simulink model "mathModel_v1"  (R2026a)
settings: Solver=VariableStepAuto  StopTime=40
InitFcn:
  | skidpad_init
undefined symbols (not defined in the file): ctrl, ic, skidpad, waypoints
libraries: slpidlib x2, sl_discontinuities x1
settings Model: Creator=lholliday  LastModifiedBy=lholliday

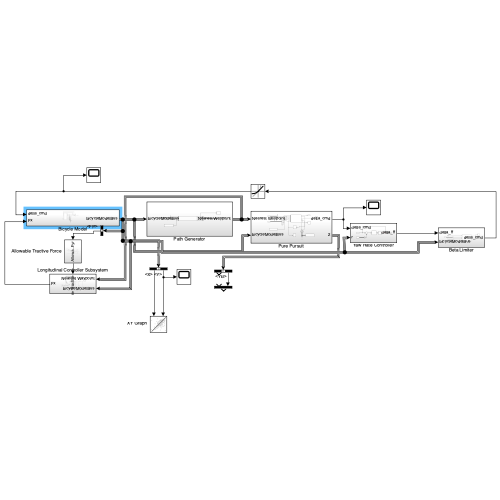
[thumbnail: Simulink's stored preview of the top-level diagram]
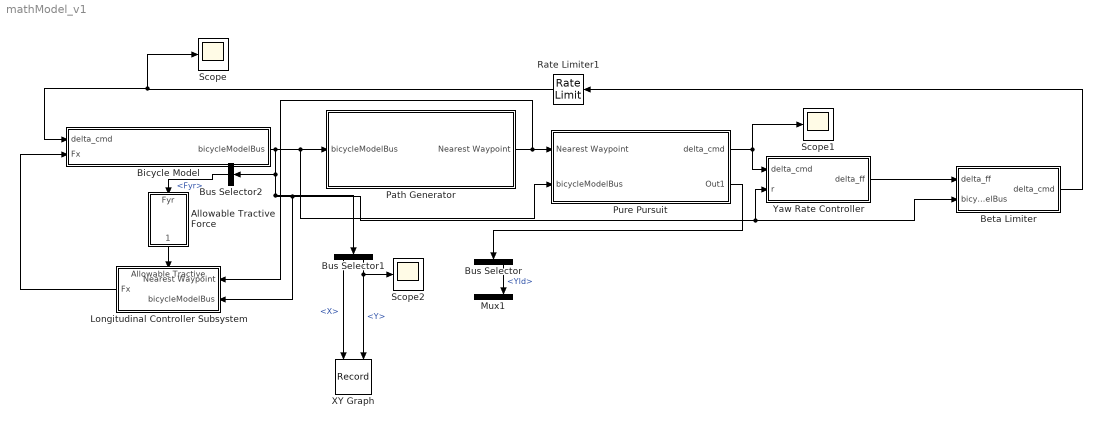
== system mathModel_v1 ==
  Allowable Tractive Force : Subsystem
  Beta Limiter : Subsystem
  Bicycle Model : Subsystem
  Bus Selector : BusSelector  OutputSignals=Xld,Yld
  Bus Selector1 : BusSelector  OutputSignals=X,Y
  Bus Selector2 : BusSelector  OutputSignals=Fyr
  Longitudinal Controller Subsystem : Subsystem
      settings: PortSchema="{\"entries\":[{\"content\":{\"sides\":[{\"content\":{\"connectorIds\":[\"In1\",\"In2\"]},\"type\":\"ConnectorPlacement.EquallySpacedRectSide\",\"uuid\":\"bfc4df2a-5cef-4a02-bb43-7ec6f11f5372\"},{\"content\":{\"connectorIds\":[\"Out1\"],\"side\":\"RIGHT\"},\"type\":\"ConnectorPlacement.EquallySpacedRectSide\",\"uuid\":\"aa21c5e5-626b-425c-a734-c90a404eca5d\"},{\"content\":{\"connectorIds\":[\"In3\"],\"side\":\"TOP\"},\"type\":\"ConnectorPlacement.EquallySpacedRectSide\",\"uuid\":\"e7d9cb0b-dcbc-491d-a1d2-601b886fc6af\"}]},\"type\":\"ConnectorPlacement.EquallySpacedConnector\",\"uuid\":\"7c1271a6-ba3b-4cb7-a1ac-4d930dd7b7e0\"}],\"packageUris\":[\"http://schema.mathworks.com/mf0/Connector/R2020b\"],\"version\":\"1.0\"}"
  Mux1 : Mux  Inputs=2
  Path Generator : Subsystem
  Pure Pursuit : Subsystem
  Rate Limiter1 : RateLimiter  RisingSlewLimit=0.2  FallingSlewLimit=-0.2  SampleTimeMode=inherited
  Scope : Scope
      settings: ActiveDisplayYMinimum=-1  ActiveDisplayYMaximum=1  DataLoggingVariableName=ScopeData8
  Scope1 : Scope
      settings: ActiveDisplayYMinimum=-1.3364775966231448  ActiveDisplayYMaximum=1.4581321408819214  DataLoggingVariableName=ScopeData9
  Scope2 : Scope
      settings: DataLoggingVariableName=ScopeData13
  XY Graph : Record  NumPorts=2.0  FileSettingsInternal="{\"entries\":[{\"content\":{\"excelSettings\":{\"content\":{},\"type\":\"Streamout.ExcelSettings\"},\"parquetSettings\":{\"content\":{},\"type\":\"Streamout.ParquetSettings\"}},\"type\":\"Streamout.FileSettingStorage\",\"uuid\":\"\"}],\"packageUris\":[\"http:\\/\\/schema.mathworks.com\\/mf0\\/streamout_blocks\\/R2020a\"],\"version\":\"1.0\"}"  FrameSettings=[0, 0]  Layout=[1 1]  SignalsInternal="{\"entries\":[{\"content\":{\"signals\":[{\"content\":{\"blockPath\":[],\"dimensions\":[1],\"domain\":\"\",\"lineColor\":\"#a2142f\",\"plots\":[ 1 ],\"port\":1,\"signalID\":1,\"signalName\":\"<X>\"},\"type\":\"RecordBlkView.Signal\",\"uuid\":\"\"},{\"content\":{\"blockPath\":[],\"dimensions\":[1],\"domain\":\"\",\"lineColor\":\"#139fff\",\"plots\":[ 1 ],\"port\":2,\"signalID\":2,\"signalName\":\"<Y>\"},\"type\":\"RecordBlkView.Signal\",\"uuid\":\"\"}]},\"type\":\"RecordBlkView.InputSignals\",\"uuid\":\"\"}],\"packageUris\":[\"http:\\/\\/schema.mathworks.com\\/mf0\\/streamout_blocks\\/R2020a\"],\"version\":\"1.0\"}"  VisualizationBindings="{\"xyplotplugin\":{\"info\":[{\"series\":[{\"bindingParametersList\":[{\"parameter\":\"X-Axis\",\"signalID\":1,\"signalName\":\"<X>\"},{\"parameter\":\"Y-Axis\",\"signalID\":2,\"signalName\":\"<Y>\"}],\"seriesID\":0}],\"subplotID\":1}]}}"  CompatibilityTag=XY
  Yaw Rate Controller : Subsystem
  wires:
  Path Generator/1(Nearest Waypoint) -> Longitudinal Controller Subsystem/1(Nearest Waypoint), Pure Pursuit/1(Nearest Waypoint)
  Bicycle Model/1(bicycleModelBus) -> Path Generator/1(bicycleModelBus), Pure Pursuit/2(bicycleModelBus), Longitudinal Controller Subsystem/2(bicycleModelBus), Beta Limiter/2(bicycleModelBus), Yaw Rate Controller/2(r), Bus Selector1/1, Bus Selector2/1
  Beta Limiter/1(delta_cmd) -> Rate Limiter1/1
  Longitudinal Controller Subsystem/1(Fx) -> Bicycle Model/2(Fx)
  Pure Pursuit/1(delta_cmd) -> Yaw Rate Controller/1(delta_cmd), Scope1/1
  Yaw Rate Controller/1(delta_ff) -> Beta Limiter/1(delta_ff)
  Pure Pursuit/2(Out1) -> Bus Selector/1
  Bus Selector/2 -> Mux1/2  "<Yld>"
  Bus Selector1/1 -> XY Graph/1  "<X>"
  Bus Selector1/2 -> Scope2/1, XY Graph/2  "<Y>"
  Rate Limiter1/1 -> Scope/1, Bicycle Model/1(delta_cmd)
  Allowable Tractive Force/1(Allowable Tractive) -> Longitudinal Controller Subsystem/3(Allowable Tractive)
  Bus Selector2/1 -> Allowable Tractive Force/1(Fyr)  "<Fyr>"

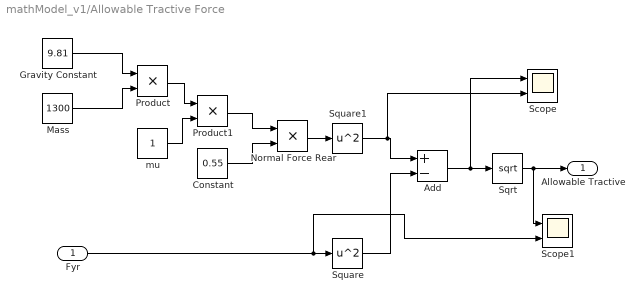
== system mathModel_v1/Allowable Tractive Force ==
  Fyr : Inport
  Add : Sum  Inputs=+-
  Constant : Constant  Value=0.55
  Gravity Constant : Constant  Value=9.81
  Mass : Constant  Value=1300
  Normal Force Rear : Product
  Product : Product
  Product1 : Product
  Scope : Scope  NumInputPorts=2
      settings: ActiveDisplayYMinimum=-2.6445905173405474E+6  ActiveDisplayYMaximum=5.4958621415815629E+7  DataLoggingVariableName=ScopeData17
  Scope1 : Scope  NumInputPorts=2
      settings: ActiveDisplayYMinimum=1109.0174008180957  ActiveDisplayYMaximum=7670.2758443535458  DataLoggingVariableName=ScopeData18
  Sqrt : Sqrt
  Square : Math  Operator=square
  Square1 : Math  Operator=square
  mu : Constant
  Allowable Tractive : Outport
  wires:
  Fyr/1 -> Scope1/2, Square/1
  Mass/1 -> Product/2
  Gravity Constant/1 -> Product/1
  mu/1 -> Product1/2
  Product/1 -> Product1/1
  Constant/1 -> Normal Force Rear/2
  Product1/1 -> Normal Force Rear/1
  Square/1 -> Add/2
  Normal Force Rear/1 -> Square1/1
  Square1/1 -> Scope/2, Add/1
  Add/1 -> Scope/1, Sqrt/1
  Sqrt/1 -> Scope1/1, Allowable Tractive/1

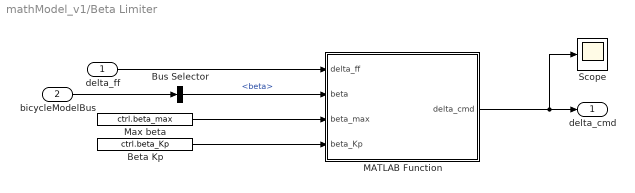
== system mathModel_v1/Beta Limiter ==
  delta_ff : Inport
  bicycleModelBus : Inport  Port=2
  Beta Kp : Constant  Value=ctrl.beta_Kp
  Bus Selector : BusSelector  OutputSignals=beta
  MATLAB Function : MATLAB Function  TreatAsAtomicUnit=on
  Max beta : Constant  Value=ctrl.beta_max
  Scope : Scope
      settings: ActiveDisplayYMinimum=-1.1215665093165463  ActiveDisplayYMaximum=1.1329055665670569  DataLoggingVariableName=ScopeData11
  delta_cmd : Outport
  wires:
  bicycleModelBus/1 -> Bus Selector/1
  delta_ff/1 -> MATLAB Function/1(delta_ff)
  Bus Selector/1 -> MATLAB Function/2(beta)  "<beta>"
  MATLAB Function/1(delta_cmd) -> delta_cmd/1, Scope/1
  Max beta/1 -> MATLAB Function/3(beta_max)
  Beta Kp/1 -> MATLAB Function/4(beta_Kp)

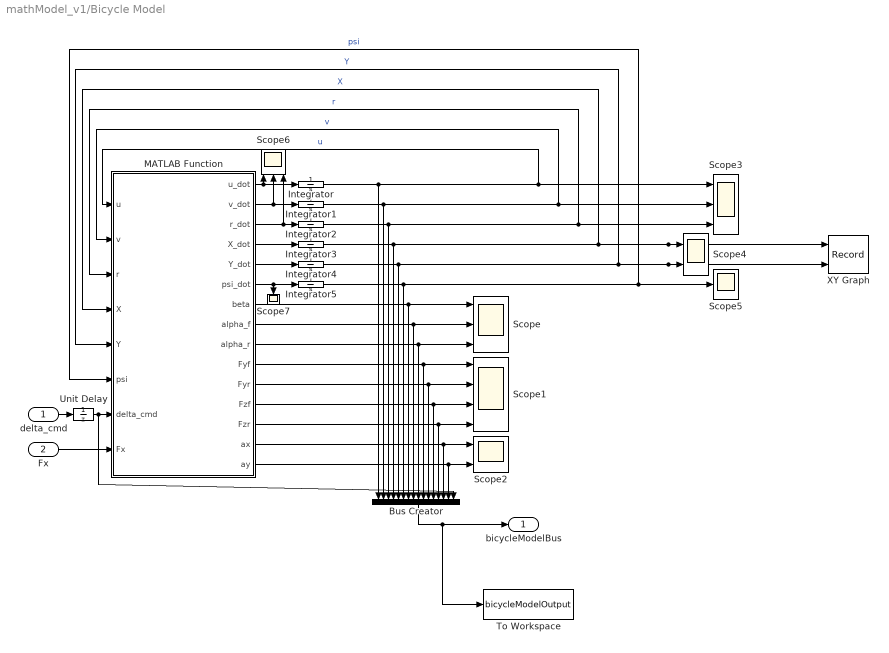
== system mathModel_v1/Bicycle Model ==
  delta_cmd : Inport
  Fx : Inport  Port=2
  Bus Creator : BusCreator  Inputs=16
  Integrator : Integrator  InitialCondition=1
  Integrator1 : Integrator
  Integrator2 : Integrator
  Integrator3 : Integrator  InitialCondition=ic.X
  Integrator4 : Integrator  InitialCondition=ic.Y
  Integrator5 : Integrator
  MATLAB Function : MATLAB Function  TreatAsAtomicUnit=on
  Scope : Scope  NumInputPorts=3
      settings: ActiveDisplayYMinimum=-3.8834487978477066  ActiveDisplayYMaximum=5.2081564111480709
  Scope1 : Scope  NumInputPorts=4
      settings: ActiveDisplayYMinimum=-1  ActiveDisplayYMaximum=1
  Scope2 : Scope  NumInputPorts=2
      settings: ActiveDisplayYMinimum=-1  ActiveDisplayYMaximum=1  DataLoggingVariableName=ScopeData2
  Scope3 : Scope  NumInputPorts=3
      settings: ActiveDisplayYMinimum=-3.5254490278371251  ActiveDisplayYMaximum=31.729041250534134  DataLoggingVariableName=ScopeData3
  Scope4 : Scope  NumInputPorts=2
      settings: ActiveDisplayYMinimum=-1031.663648785918  ActiveDisplayYMaximum=2103.4580897021219  DataLoggingVariableName=ScopeData4
  Scope5 : Scope
      settings: ActiveDisplayYMinimum=-1  ActiveDisplayYMaximum=1  DataLoggingVariableName=ScopeData5
  Scope6 : Scope  NumInputPorts=3
      settings: ActiveDisplayYMinimum=-1.4708935468625282  ActiveDisplayYMaximum=6.1584326163180583  DataLoggingVariableName=ScopeData6
  Scope7 : Scope
      settings: ActiveDisplayYMinimum=-1.109696536806452  ActiveDisplayYMaximum=1.2916224827655673  DataLoggingVariableName=ScopeData10
  To Workspace : ToWorkspace  VariableName=bicycleModelOutput  SaveFormat=Timeseries  SampleTime=-1
  Unit Delay : UnitDelay  SampleTime=-1
  XY Graph : Record  NumPorts=2.0  FileSettingsInternal="{\"entries\":[{\"content\":{\"excelSettings\":{\"content\":{},\"type\":\"Streamout.ExcelSettings\"},\"parquetSettings\":{\"content\":{},\"type\":\"Streamout.ParquetSettings\"}},\"type\":\"Streamout.FileSettingStorage\",\"uuid\":\"\"}],\"packageUris\":[\"http:\\/\\/schema.mathworks.com\\/mf0\\/streamout_blocks\\/R2020a\"],\"version\":\"1.0\"}"  FrameSettings=[0, 0]  Layout=[1 1]  SignalsInternal="{\"entries\":[{\"content\":{\"signals\":[{\"content\":{\"blockPath\":[],\"dimensions\":[1],\"domain\":\"\",\"lineColor\":\"#a2142f\",\"plots\":[ 1 ],\"port\":1,\"signalID\":1,\"signalName\":\"X\"},\"type\":\"RecordBlkView.Signal\",\"uuid\":\"\"},{\"content\":{\"blockPath\":[],\"dimensions\":[1],\"domain\":\"\",\"lineColor\":\"#139fff\",\"plots\":[ 1 ],\"port\":2,\"signalID\":2,\"signalName\":\"Y\"},\"type\":\"RecordBlkView.Signal\",\"uuid\":\"\"}]},\"type\":\"RecordBlkView.InputSignals\",\"uuid\":\"\"}],\"packageUris\":[\"http:\\/\\/schema.mathworks.com\\/mf0\\/streamout_blocks\\/R2020a\"],\"version\":\"1.0\"}"  VisualizationBindings="{\"xyplotplugin\":{\"info\":[{\"series\":[{\"bindingParametersList\":[{\"parameter\":\"X-Axis\",\"signalID\":1,\"signalName\":\"X\"},{\"parameter\":\"Y-Axis\",\"signalID\":2,\"signalName\":\"Y\"}],\"seriesID\":0}],\"subplotID\":1}]}}"  CompatibilityTag=XY
  bicycleModelBus : Outport
  wires:
  ? -> ?
  MATLAB Function/2(v_dot) -> Scope6/2, Integrator1/1
  MATLAB Function/3(r_dot) -> Scope6/3, Integrator2/1
  MATLAB Function/4(X_dot) -> Integrator3/1
  MATLAB Function/5(Y_dot) -> Integrator4/1
  MATLAB Function/6(psi_dot) -> Scope7/1, Integrator5/1
  MATLAB Function/1(u_dot) -> Scope6/1, Integrator/1
  Integrator1/1 -> Scope3/2, MATLAB Function/2(v), Bus Creator/2  "v"
  Integrator2/1 -> Scope3/3, MATLAB Function/3(r), Bus Creator/3  "r"
  Integrator3/1 -> MATLAB Function/4(X), XY Graph/1, Scope4/1, Bus Creator/4  "X"
  Integrator4/1 -> MATLAB Function/5(Y), XY Graph/2, Scope4/2, Bus Creator/5  "Y"
  Integrator5/1 -> MATLAB Function/6(psi), Scope5/1, Bus Creator/6  "psi"
  MATLAB Function/8(alpha_f) -> Scope/2, Bus Creator/8
  MATLAB Function/7(beta) -> Scope/1, Bus Creator/7
  MATLAB Function/9(alpha_r) -> Scope/3, Bus Creator/9
  MATLAB Function/10(Fyf) -> Scope1/1, Bus Creator/10
  MATLAB Function/11(Fyr) -> Scope1/2, Bus Creator/11
  MATLAB Function/12(Fzf) -> Scope1/3, Bus Creator/12
  MATLAB Function/13(Fzr) -> Scope1/4, Bus Creator/13
  MATLAB Function/15(ay) -> Scope2/2, Bus Creator/15
  MATLAB Function/14(ax) -> Scope2/1, Bus Creator/14
  Fx/1 -> MATLAB Function/8(Fx)
  Bus Creator/1 -> To Workspace/1, bicycleModelBus/1
  Integrator/1 -> Scope3/1, MATLAB Function/1(u), Bus Creator/1  "u"
  delta_cmd/1 -> Unit Delay/1
  Unit Delay/1 -> Bus Creator/16, MATLAB Function/7(delta_cmd)

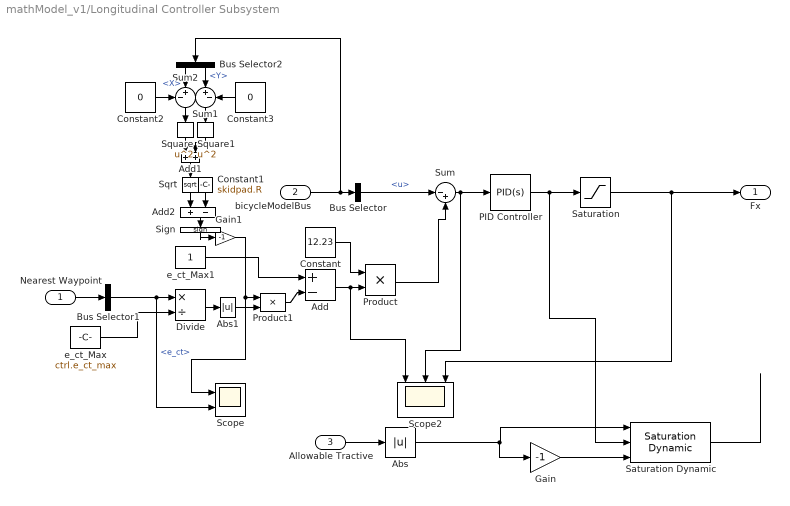
== system mathModel_v1/Longitudinal Controller Subsystem ==
  Nearest Waypoint : Inport
  bicycleModelBus : Inport  Port=2
  Allowable Tractive : Inport  Port=3
  Abs : Abs  SaturateOnIntegerOverflow=off
  Abs1 : Abs  SaturateOnIntegerOverflow=off
  Add : Sum  Inputs=+-
  Add1 : Sum
  Add2 : Sum  Inputs=+-
  Bus Selector : BusSelector  OutputSignals=u
  Bus Selector1 : BusSelector  OutputSignals=e_ct
  Bus Selector2 : BusSelector  OutputSignals=X,Y
  Constant : Constant  Value=12.23
  Constant1 : Constant  Value=skidpad.R
  Constant2 : Constant  Value=0
  Constant3 : Constant  Value=0
  Divide : Product  Inputs=*/
  Gain : Gain  Gain=-1
  Gain1 : Gain  Gain=-1
  PID Controller : slpidlib/PID Controller  Controller=PID  Form=Parallel  TimeDomain=Continuous-time  UseExternalTs=off  SampleTime=-1  IntegratorMethod=Forward Euler  FilterMethod=Forward Euler  ControllerParametersSource=internal  P=ctrl.spd_Kp  I=ctrl.spd_Ki  UseKiTs=off  D=ctrl.spd_Kd  UseExternalDerivativeSource=off  N=100  UseFilter=on  TunerSelectOption=Transfer Function Based (PID Tuner App)  InitialConditionSource=internal  InitialConditionForIntegrator=0  InitialConditionForFilter=0  DifferentiatorICPrevScaledInput=0  ExternalReset=none  TrackingMode=off  Kt=1  LimitOutput=off  SatLimitsSource=internal  UpperSaturationLimit=inf  LowerSaturationLimit=-inf  LinearizeAsGain=on  AntiWindupMode=none  Kb=1  LimitIntegrator=off  UpperIntegratorSaturationLimit=inf  LowerIntegratorSaturationLimit=-inf  POutMin=[]  POutMax=[]  IOutMin=[]  IOutMax=[]  DOutMin=[]  DOutMax=[]  NOutMin=[]  NOutMax=[]  SumOutMin=[]  SumOutMax=[]  SaturationOutMin=[]  SaturationOutMax=[]  PParamMin=[]  PParamMax=[]  IParamMin=[]  IParamMax=[]  DParamMin=[]  DParamMax=[]  NParamMin=[]  NParamMax=[]  KbParamMin=[]  KbParamMax=[]  KtParamMin=[]  KtParamMax=[]  KbOutMin=[]  KbOutMax=[]  KtOutMin=[]  KtOutMax=[]  IntegratorOutMin=[]  IntegratorOutMax=[]  FilterOutMin=[]  FilterOutMax=[]  SumI1OutMin=[]  SumI1OutMax=[]  SumI2OutMin=[]  SumI2OutMax=[]  SumI3OutMin=[]  SumI3OutMax=[]  SumI4OutMin=[]  SumI4OutMax=[]  SumDOutMin=[]  SumDOutMax=[]  DifferentiatorOutMin=[]  DifferentiatorOutMax=[]  FilterDiffOutCoefMin=[]  FilterDiffOutCoefMax=[]  ReciprocalOutMin=[]  ReciprocalOutMax=[]  SumDenOutMin=[]  SumDenOutMax=[]  SumNumOutMin=[]  SumNumOutMax=[]  DivideOutMin=[]  DivideOutMax=[]  UdiffTsProdOutMin=[]  UdiffTsProdOutMax=[]  NTsProdOutMin=[]  NTsProdOutMax=[]  UintegralTsProdOutMin=[]  UintegralTsProdOutMax=[]  UngainTsProdOutMin=[]  UngainTsProdOutMax=[]  ClampingZeroOutDataTypeStr=Inherit: Inherit via back propagation  ClampingZeroOutMin=[]  ClampingZeroOutMax=[]  FilterDenConstantOutDataTypeStr=Inherit: Inherit via back propagation  FilterDenConstantOutMin=[]  FilterDenConstantOutMax=[]  PCopyOutDataTypeStr=Inherit: Inherit via back propagation  PCopyOutMin=[]  PCopyOutMax=[]  NCopyOutDataTypeStr=Inherit: Inherit via back propagation  NCopyOutMin=[]  NCopyOutMax=[]  IntegratorContinuousStateAttributes=''  IntegratorStateMustResolveToSignalObject=off  IntegratorRTWStateStorageClass=Auto  FilterContinuousStateAttributes=''  FilterStateMustResolveToSignalObject=off  FilterRTWStateStorageClass=Auto  ParallelPVariant=InternalParameters  IdealPVariant=Disabled  IVariant=InternalParameters  DVariant=InternalParameters  IntegratorVariant=Continuous  SatVariant=Disabled  AWVariant=Passthrough  PCopyVariant=Disabled  TRVariant=Disabled  FdbkBlocksVariant=Forward  IdealPFdbkVariant=Disabled  SatFdbkVariant=Disabled  DerivativeFilterVariant=ContFilter  NVariant=InternalParameters  NCopyVariant=Disabled  FilterICVariant=InternalICsFilter  IntegratorICVariant=InternalICs  ExternalResetVariant=Disabled  TRSumVariant=Passthrough  SumFdbkVariant=Disabled  SumVariant=Sum_PID  TsampFilterVariant=InternalTs  TsampNgainVariant=Passthrough  TsampIntegralVariant=Disabled_SignalSpec  ExternalSaturationOutDataTypeStr=Inherit: Same as second input  DerivativeSourceVariant=ErrorSignal  PreIntVariant=InternalPreInt
  Product : Product
  Product1 : Product
  Saturation : Saturate  UpperLimit=ctrl.Fx_max  LowerLimit=ctrl.Fx_min
  Saturation Dynamic : sl_discontinuities/Saturation Dynamic  OutMin=[]  OutMax=[]  OutDataTypeStr=Inherit: Same as second input  OutDataType=fixdt(1, 16)  OutScaling=2^-10  DoSatur=off
      settings: LibrarySourceBlock=|
      | simulink/Discontinuities/Saturation
      | Dynamic
  Scope : Scope  NumInputPorts=2
      settings: ActiveDisplayYMinimum=-48.92468742696137  ActiveDisplayYMaximum=48.607667503868036  DataLoggingVariableName=ScopeData16
  Scope2 : Scope  NumInputPorts=3
      settings: ActiveDisplayYMinimum=-0.082162988080077839  ActiveDisplayYMaximum=1.1202403320088976  DataLoggingVariableName=ScopeData19
  Sign : Signum
  Sqrt : Sqrt
  Square : Math  Operator=square
  Square1 : Math  Operator=square
  Sum : Sum  Inputs=|-+
  Sum1 : Sum  Inputs=|+-
  Sum2 : Sum  Inputs=-+|
  e_ct_Max : Constant  Value=ctrl.e_ct_max
  e_ct_Max1 : Constant
  Fx : Outport
  wires:
  bicycleModelBus/1 -> Bus Selector/1, Bus Selector2/1
  Sum/1 -> PID Controller/1, Scope2/2
  PID Controller/1 -> Saturation/1, Saturation Dynamic/2
  Saturation/1 -> Scope2/3, Fx/1
  Allowable Tractive/1 -> Abs/1
  Abs/1 -> Gain/1, Saturation Dynamic/1
  Gain/1 -> Saturation Dynamic/3
  Saturation Dynamic/1 -> ?
  Nearest Waypoint/1 -> Bus Selector1/1
  Bus Selector1/1 -> Scope/2, Divide/1  "<e_ct>"
  e_ct_Max/1 -> Divide/2
  Divide/1 -> Abs1/1
  Product/1 -> Sum/2
  e_ct_Max1/1 -> Add/1
  Add/1 -> Scope2/1, Product/2
  Bus Selector/1 -> Sum/1  "<u>"
  Constant/1 -> Product/1
  Square/1 -> Add1/1
  Square1/1 -> Add1/2
  Add1/1 -> Sqrt/1
  Sqrt/1 -> Add2/1
  Constant1/1 -> Add2/2
  Add2/1 -> Sign/1
  Abs1/1 -> Product1/2
  Sign/1 -> Gain1/1
  Product1/1 -> Add/2
  Constant3/1 -> Sum1/2
  Bus Selector2/2 -> Sum1/1  "<Y>"
  Sum1/1 -> Square1/1
  Sum2/1 -> Square/1
  Bus Selector2/1 -> Sum2/2  "<X>"
  Constant2/1 -> Sum2/1
  Gain1/1 -> Scope/1, Product1/1

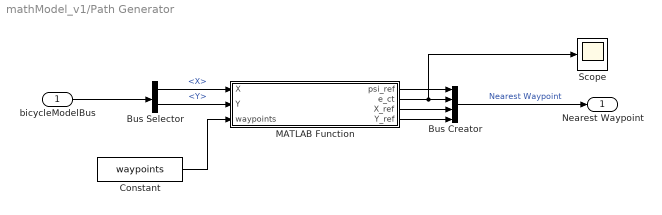
== system mathModel_v1/Path Generator ==
  bicycleModelBus : Inport
  Bus Creator : BusCreator  Inputs=4
  Bus Selector : BusSelector  OutputSignals=X,Y
  Constant : Constant  Value=waypoints
  MATLAB Function : MATLAB Function  TreatAsAtomicUnit=on
  Scope : Scope
      settings: ActiveDisplayYMinimum=-362.12936641992621  ActiveDisplayYMaximum=253.81612411681579  DataLoggingVariableName=ScopeData7
  Nearest Waypoint : Outport
  wires:
  bicycleModelBus/1 -> Bus Selector/1
  Bus Selector/1 -> MATLAB Function/1(X)  "<X>"
  Bus Selector/2 -> MATLAB Function/2(Y)  "<Y>"
  MATLAB Function/1(psi_ref) -> Bus Creator/1
  MATLAB Function/2(e_ct) -> Scope/1, Bus Creator/2
  MATLAB Function/3(X_ref) -> Bus Creator/3
  MATLAB Function/4(Y_ref) -> Bus Creator/4
  Bus Creator/1 -> Nearest Waypoint/1  "Nearest Waypoint"
  Constant/1 -> MATLAB Function/3(waypoints)

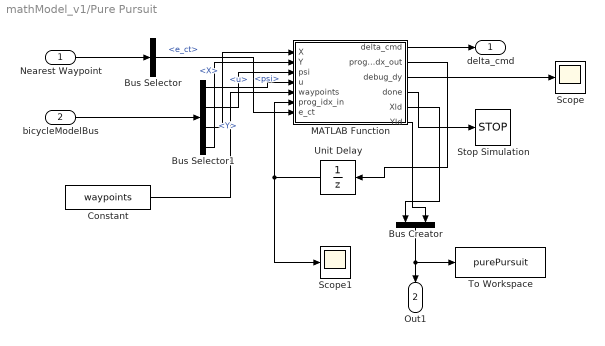
== system mathModel_v1/Pure Pursuit ==
  Nearest Waypoint : Inport
  bicycleModelBus : Inport  Port=2
  Bus Creator : BusCreator  Inputs=2
  Bus Selector : BusSelector  OutputSignals=e_ct
  Bus Selector1 : BusSelector  OutputSignals=u,psi,X,Y
  Constant : Constant  Value=waypoints
  MATLAB Function : MATLAB Function  TreatAsAtomicUnit=on
  Scope : Scope
      settings: ActiveDisplayYMinimum=-282.00787938495415  ActiveDisplayYMaximum=340.50274168342952  DataLoggingVariableName=ScopeData12
  Scope1 : Scope
      settings: ActiveDisplayYMinimum=-19.874999999999996  ActiveDisplayYMaximum=188.875  DataLoggingVariableName=ScopeData14
  Stop Simulation : Stop
  To Workspace : ToWorkspace  VariableName=purePursuit  SaveFormat=Timeseries  SampleTime=-1
  Unit Delay : UnitDelay  InitialCondition=1  SampleTime=0.01
  delta_cmd : Outport
  Out1 : Outport  Port=2
  wires:
  bicycleModelBus/1 -> Bus Selector1/1
  Nearest Waypoint/1 -> Bus Selector/1
  Bus Selector1/1 -> MATLAB Function/4(u)  "<u>"
  Bus Selector1/2 -> MATLAB Function/3(psi)  "<psi>"
  MATLAB Function/1(delta_cmd) -> delta_cmd/1
  Bus Selector1/3 -> MATLAB Function/1(X)  "<X>"
  Bus Selector1/4 -> MATLAB Function/2(Y)  "<Y>"
  Constant/1 -> MATLAB Function/5(waypoints)
  MATLAB Function/3(debug_dy) -> Scope/1
  MATLAB Function/2(prog_idx_out) -> Unit Delay/1
  Unit Delay/1 -> MATLAB Function/6(prog_idx_in), Scope1/1
  MATLAB Function/4(done) -> Stop Simulation/1
  Bus Creator/1 -> To Workspace/1, Out1/1
  MATLAB Function/5(Xld) -> Bus Creator/1
  MATLAB Function/6(Yld) -> Bus Creator/2
  Bus Selector/1 -> MATLAB Function/7(e_ct)  "<e_ct>"

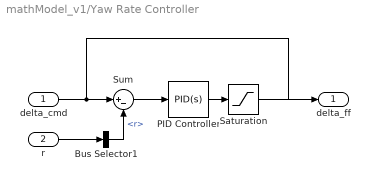
== system mathModel_v1/Yaw Rate Controller ==
  delta_cmd : Inport
  r : Inport  Port=2
  Bus Selector1 : BusSelector  OutputSignals=r
  PID Controller : slpidlib/PID Controller  Controller=PID  Form=Parallel  TimeDomain=Continuous-time  UseExternalTs=off  SampleTime=-1  IntegratorMethod=Forward Euler  FilterMethod=Forward Euler  ControllerParametersSource=internal  P=0.3  I=0.05  UseKiTs=off  D=0  UseExternalDerivativeSource=off  N=100  UseFilter=on  TunerSelectOption=Transfer Function Based (PID Tuner App)  InitialConditionSource=internal  InitialConditionForIntegrator=0  InitialConditionForFilter=0  DifferentiatorICPrevScaledInput=0  ExternalReset=none  TrackingMode=off  Kt=1  LimitOutput=off  SatLimitsSource=internal  UpperSaturationLimit=inf  LowerSaturationLimit=-inf  LinearizeAsGain=on  AntiWindupMode=none  Kb=1  LimitIntegrator=off  UpperIntegratorSaturationLimit=inf  LowerIntegratorSaturationLimit=-inf  POutMin=[]  POutMax=[]  IOutMin=[]  IOutMax=[]  DOutMin=[]  DOutMax=[]  NOutMin=[]  NOutMax=[]  SumOutMin=[]  SumOutMax=[]  SaturationOutMin=[]  SaturationOutMax=[]  PParamMin=[]  PParamMax=[]  IParamMin=[]  IParamMax=[]  DParamMin=[]  DParamMax=[]  NParamMin=[]  NParamMax=[]  KbParamMin=[]  KbParamMax=[]  KtParamMin=[]  KtParamMax=[]  KbOutMin=[]  KbOutMax=[]  KtOutMin=[]  KtOutMax=[]  IntegratorOutMin=[]  IntegratorOutMax=[]  FilterOutMin=[]  FilterOutMax=[]  SumI1OutMin=[]  SumI1OutMax=[]  SumI2OutMin=[]  SumI2OutMax=[]  SumI3OutMin=[]  SumI3OutMax=[]  SumI4OutMin=[]  SumI4OutMax=[]  SumDOutMin=[]  SumDOutMax=[]  DifferentiatorOutMin=[]  DifferentiatorOutMax=[]  FilterDiffOutCoefMin=[]  FilterDiffOutCoefMax=[]  ReciprocalOutMin=[]  ReciprocalOutMax=[]  SumDenOutMin=[]  SumDenOutMax=[]  SumNumOutMin=[]  SumNumOutMax=[]  DivideOutMin=[]  DivideOutMax=[]  UdiffTsProdOutMin=[]  UdiffTsProdOutMax=[]  NTsProdOutMin=[]  NTsProdOutMax=[]  UintegralTsProdOutMin=[]  UintegralTsProdOutMax=[]  UngainTsProdOutMin=[]  UngainTsProdOutMax=[]  ClampingZeroOutDataTypeStr=Inherit: Inherit via back propagation  ClampingZeroOutMin=[]  ClampingZeroOutMax=[]  FilterDenConstantOutDataTypeStr=Inherit: Inherit via back propagation  FilterDenConstantOutMin=[]  FilterDenConstantOutMax=[]  PCopyOutDataTypeStr=Inherit: Inherit via back propagation  PCopyOutMin=[]  PCopyOutMax=[]  NCopyOutDataTypeStr=Inherit: Inherit via back propagation  NCopyOutMin=[]  NCopyOutMax=[]  IntegratorContinuousStateAttributes=''  IntegratorStateMustResolveToSignalObject=off  IntegratorRTWStateStorageClass=Auto  FilterContinuousStateAttributes=''  FilterStateMustResolveToSignalObject=off  FilterRTWStateStorageClass=Auto  ParallelPVariant=InternalParameters  IdealPVariant=Disabled  IVariant=InternalParameters  DVariant=InternalParameters  IntegratorVariant=Continuous  SatVariant=Disabled  AWVariant=Passthrough  PCopyVariant=Disabled  TRVariant=Disabled  FdbkBlocksVariant=Forward  IdealPFdbkVariant=Disabled  SatFdbkVariant=Disabled  DerivativeFilterVariant=ContFilter  NVariant=InternalParameters  NCopyVariant=Disabled  FilterICVariant=InternalICsFilter  IntegratorICVariant=InternalICs  ExternalResetVariant=Disabled  TRSumVariant=Passthrough  SumFdbkVariant=Disabled  SumVariant=Sum_PID  TsampFilterVariant=InternalTs  TsampNgainVariant=Passthrough  TsampIntegralVariant=Disabled_SignalSpec  ExternalSaturationOutDataTypeStr=Inherit: Same as second input  DerivativeSourceVariant=ErrorSignal  PreIntVariant=InternalPreInt
  Saturation : Saturate  UpperLimit=30*pi()/180  LowerLimit=- 30*pi()/180
  Sum : Sum  Inputs=|+-
  delta_ff : Outport
  wires:
  r/1 -> Bus Selector1/1
  Sum/1 -> PID Controller/1
  Bus Selector1/1 -> Sum/2  "<r>"
  PID Controller/1 -> Saturation/1
  Saturation/1 -> ?
  delta_cmd/1 -> delta_ff/1, Sum/1

== matlab function mathModel_v1/Path Generator/MATLAB Function ==
  data: X input; psi_ref output; Y input; e_ct output; X_ref output; Y_ref output; waypoints input
function [psi_ref, e_ct, X_ref, Y_ref] = nearest_waypoint(X, Y, waypoints)

% Find nearest waypoint
dx   = waypoints(:,1) - X;
dy   = waypoints(:,2) - Y;
dist = sqrt(dx.^2 + dy.^2);
[~, idx] = min(dist);

psi_ref = waypoints(idx, 3);
X_ref   = waypoints(idx, 1);
Y_ref   = waypoints(idx, 2);

dx_ref = X - X_ref;
dy_ref = Y - Y_ref;
e_ct   = -sin(psi_ref)*dx_ref + cos(psi_ref)*dy_ref;

== matlab function mathModel_v1/Bicycle Model/MATLAB Function ==
  data: u_dot output; v_dot output; u input; v input; r_dot output; X_dot output; r input; X input; Y input; psi input; delta_cmd input; Fx input; Y_dot output; psi_dot output; beta output; alpha_f output; alpha_r output; Fyf output; Fyr output; Fzf output; Fzr output; ax output; ay output
function [u_dot, v_dot, r_dot, X_dot, Y_dot, psi_dot, ...
          beta, alpha_f, alpha_r, Fyf, Fyr, Fzf, Fzr, ax, ay] = ...
    bicycle_model_plant(u, v, r, X, Y, psi, delta_cmd, Fx)

% BICYCLE_MODEL_PLANT Nonlinear 6-DOF bicycle model with Pacejka tyres.
%
% INPUTS:
%   u         - Longitudinal velocity [m/s]
%   v         - Lateral velocity [m/s]
%   r         - Yaw rate [rad/s]
%   X, Y      - Global position [m]
%   psi       - Heading [rad]
%   delta_cmd - Front wheel steer angle [rad]
%   Fx        - Longitudinal force at rear axle [N]
%
% OUTPUTS:
%   u_dot, v_dot, r_dot     - Derivatives of velocities [m/s^2, rad/s^2]
%   X_dot, Y_dot, psi_dot   - Derivatives of position and heading
%   beta                     - Body slip angle [rad]
%   alpha_f, alpha_r         - Front and rear slip angles [rad]
%   Fyf, Fyr                 - Front and rear lateral tyre forces [N]
%   Fzf, Fzr                 - Front and rear normal loads [N]
%   ax, ay                   - Longitudinal and lateral accelerations [m/s^2]

% Load vehicle and tyre parameters from base workspace
% veh  = evalin('base', 'veh');
% tyre = evalin('base', 'tyre');


veh.m    = 1300;        % Total mass [kg]
veh.L    = 2.750;       % Wheelbase [m]
veh.a    = 1.468;       % CG to front axle [m]
veh.b    = 2.750 - 1.468; % CG to rear axle [m]
veh.Iz   = 1850;        % Yaw moment of inertia [kg.m^2]
veh.h_cg = 0.45;        % CG height [m]
veh.mu   = 1.0;         % Road friction coefficient [-]
veh.g    = 9.81;        % Gravitational acceleration [m/s^2]


% Unpack vehicle parameters
m    = veh.m;       % Total mass [kg]
L    = veh.L;       % Wheelbase [m]
a    = veh.a;       % CG to front axle [m]
b    = veh.b;       % CG to rear axle [m]
Iz   = veh.Iz;      % Yaw moment of inertia [kg.m^2]
mu   = veh.mu;      % Friction coefficient [-]
g    = veh.g;       % Gravity [m/s^2]
% Front tyre

tyre.f.B = 10.0;        % Stiffness factor [-]
tyre.f.C = 1.9;         % Shape factor [-]
tyre.f.E = 0.97;        % Curvature factor [-]

% Rear tyre
tyre.r.B = 10.0;
tyre.r.C = 1.9;
tyre.r.E = 0.97;
% -------------------------------------------------------------------------
% Normal Loads (static, no roll dynamics)
% -------------------------------------------------------------------------

Fzf = m * g * b / L;    % Front axle normal load [N]
Fzr = m * g * a / L;    % Rear axle normal load [N]

% -------------------------------------------------------------------------
% Slip Angles
% -------------------------------------------------------------------------

% Guard against u near zero
u_safe = max(u, 0.1);

% Front slip angle
alpha_f = delta_cmd - atan2(v + a*r, u_safe);

% Rear slip angle
alpha_r = -atan2(v - b*r, u_safe);

% -------------------------------------------------------------------------
% Pacejka Magic Formula Lateral Tyre Forces
% -------------------------------------------------------------------------

% Front tyre
Fyf = pacejka_force(alpha_f, Fzf, tyre.f.B, tyre.f.C, tyre.f.E, mu);

% Rear tyre
Fyr = pacejka_force(alpha_r, Fzr, tyre.r.B, tyre.r.C, tyre.r.E, mu);

% -------------------------------------------------------------------------
% Equations of Motion (Body Frame)
% -------------------------------------------------------------------------

% Longitudinal: m(u_dot - v*r) = Fx - Fyf*sin(delta_cmd)
u_dot = (Fx - Fyf*sin(delta_cmd))/m + v*r;

% Lateral: m(v_dot + u*r) = Fyf*cos(delta_cmd) + Fyr
v_dot = (Fyf*cos(delta_cmd) + Fyr)/m - u*r;

% Yaw: Iz*r_dot = a*Fyf*cos(delta_cmd) - b*Fyr
r_dot = (a*Fyf*cos(delta_cmd) - b*Fyr) / Iz;

% -------------------------------------------------------------------------
% Kinematics (Global Frame)
% -------------------------------------------------------------------------

X_dot   = u*cos(psi) - v*sin(psi);
Y_dot   = u*sin(psi) + v*cos(psi);
psi_dot = r;

% -------------------------------------------------------------------------
% Body Slip Angle
% -------------------------------------------------------------------------

beta = atan2(v, u_safe);

% -------------------------------------------------------------------------
% Accelerations (for logging/monitoring)
% -------------------------------------------------------------------------

ax = u_dot;
ay = v_dot + u*r;

end

% =========================================================================
% PACEJKA_FORCE  Compute lateral tyre force from slip angle and normal load.
% =========================================================================

function Fy = pacejka_force(alpha, Fz, B, C, E, mu)
% Pure lateral Pacejka Magic Formula
%   Fy = D*sin(C*atan(B*alpha - E*(B*alpha - atan(B*alpha))))
% where D = mu*Fz (peak force)

D = mu * Fz;

% Compute atan(B*alpha) once
Balpha      = B * alpha;
arctan_Balpha = atan(Balpha);

% Argument to outer atan
inner_arg = Balpha - E * (Balpha - arctan_Balpha);

% Pacejka formula
Fy = D * sin(C * atan(inner_arg));

end

== matlab function mathModel_v1/Pure Pursuit/MATLAB Function ==
  settings: updateMethod=DISCRETE
  data: X input; Y input; psi input; u input; delta_cmd output; waypoints input; prog_idx_out output; debug_dy output; prog_idx_in input; done output; Xld output; Yld output; e_ct input
function [delta_cmd, prog_idx_out, debug_dy, done, Xld, Yld]  = pure_pursuit(X, Y, psi, u, waypoints, prog_idx_in, e_ct)

Ld     = 5.0;
L      = 2.750;
u_safe = max(u, 0.1);
n      = int32(size(waypoints, 1));

% Cast to int32
idx = int32(prog_idx_in);

% Advance index forward only
for i = idx:min(idx + int32(20), n)
    d = sqrt((waypoints(i,1) - X)^2 + (waypoints(i,2) - Y)^2);
    if d < 3.0
        idx = i;
    end
end

% Find lookahead
lookahead_idx = idx;
for i = idx:n
    d = sqrt((waypoints(i,1) - X)^2 + (waypoints(i,2) - Y)^2);
    if d >= Ld
        lookahead_idx = i;
        break;
    end
end

Xld   = waypoints(lookahead_idx, 1);
Yld   = waypoints(lookahead_idx, 2);

dx_ld =  cos(psi)*(Xld - X) + sin(psi)*(Yld - Y);
dy_ld = -sin(psi)*(Xld - X) + cos(psi)*(Yld - Y);

debug_dy  = dy_ld;
kappa     = 2*dy_ld / (Ld^2);
delta     = atan(kappa * L);
% delta     = max(min(delta, 30*pi/180), -30*pi/180);
% delta_cmd = delta;


k_ct   = 0.0;   % tunable — start small
delta  = delta + k_ct * e_ct;
delta  = max(min(delta, 20*pi/180), -20*pi/180);
prog_idx_out = double(idx);
delta_cmd = delta;
done = double(idx >= n - int32(5));

== matlab function mathModel_v1/Beta Limiter/MATLAB Function ==
  data: delta_ff input; beta input; beta_max input; beta_Kp input; delta_cmd output
function delta_cmd = beta_limiter(delta_ff, beta, beta_max, beta_Kp)

% Compute how much beta exceeds the limit (zero if within limit)
beta_err = max(0, abs(beta) - beta_max);

% Correction always opposes the sign of beta
delta_correction = -beta_Kp * sign(beta) * beta_err;

% Add correction to feedforward steer
delta_cmd = delta_ff + delta_correction;

% Clamp to steering limit
delta_cmd = max(min(delta_cmd, 30*pi/180), -30*pi/180);
